simulink model "untitled3"  (R2022b)
settings: Solver=VariableStepAuto  StartTime=0.0  StopTime=10.0  RelTol=1e-3
settings Model: Creator=admin  LastModifiedBy=admin

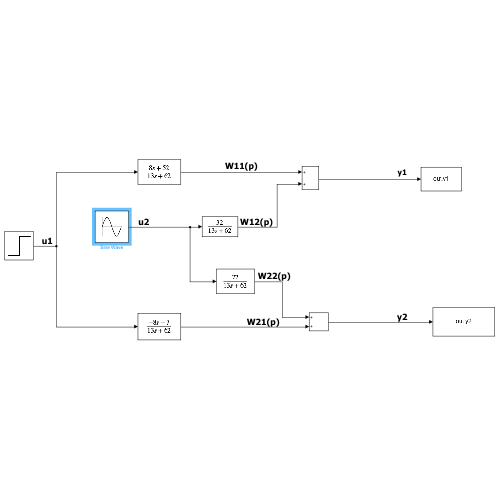
[thumbnail: Simulink's stored preview of the top-level diagram]
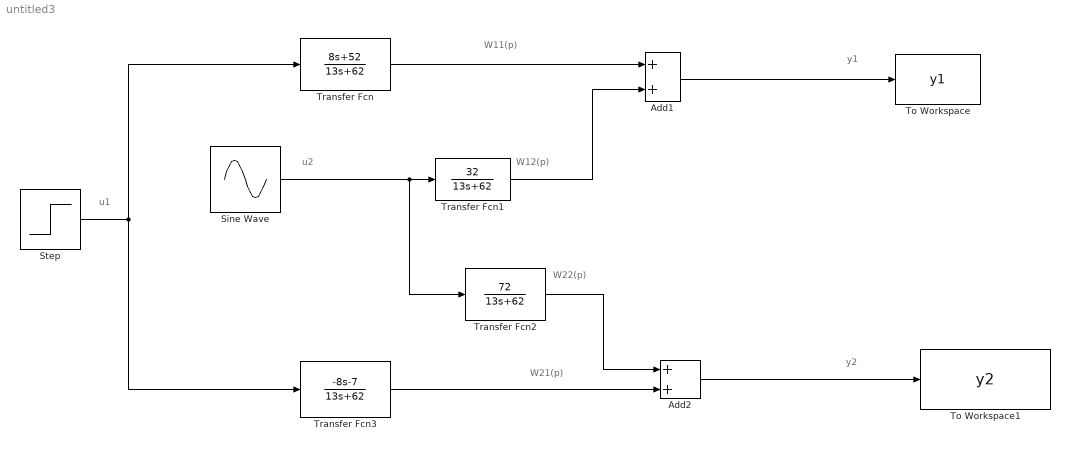
== system untitled3 ==
  note: W21(p)
  note: W22(p)
  note: W12(p)
  note: W11(p)
  note: y2
  note: y1
  note: u1
  note: u2
  Add1 : Sum
  Add2 : Sum
  Sine Wave : Sin  SampleTime=0
  Step : Step  SampleTime=0
  To Workspace : ToWorkspace  VariableName=y1  SaveFormat=Structure With Time  SampleTime=-1
  To Workspace1 : ToWorkspace  VariableName=y2  SaveFormat=Structure With Time  SampleTime=-1
  Transfer Fcn : TransferFcn  Numerator=[8 52]  Denominator=[13 62]
  Transfer Fcn1 : TransferFcn  Numerator=[0 32]  Denominator=[13 62]
  Transfer Fcn2 : TransferFcn  Numerator=[0 72]  Denominator=[13 62]
  Transfer Fcn3 : TransferFcn  Numerator=[-8 -7]  Denominator=[13 62]
  wires:
  Step/1 -> Transfer Fcn3/1, Transfer Fcn/1
  Transfer Fcn/1 -> Add1/1
  Transfer Fcn3/1 -> Add2/2
  Sine Wave/1 -> Transfer Fcn2/1, Transfer Fcn1/1
  Transfer Fcn1/1 -> Add1/2
  Transfer Fcn2/1 -> Add2/1
  Add2/1 -> To Workspace1/1
  Add1/1 -> To Workspace/1
